simulink model "joint_sim_v1"  (R2018b)
settings: Solver=FixedStepAuto  StartTime=0.0  StopTime=8  FixedStep=0.001  MaxStep=0.001  RelTol=1e-3
undefined symbols (not defined in the file): alpha, D_el, F_c, F_s, J_joint, J_load, K_el, Kd_pos, Kd_trq, Kd_zf, Kp_pos, Kp_trq, Kp_zf, Ks_pos, Ks_trq, Ks_zf, Kt_pos, Kt_trq, Kt_zf, sigbuilder_block, sigma0, sigma1, sigma2, T_cur, T_signal_LPF, tau_max_ctrl, vs, X, Y, Z
libraries: sm_lib x6, nesl_utility x3, fcnLib4joint_sim x2, simulink x1
settings Model: Creator=l.ho  LastModifiedBy=qiming

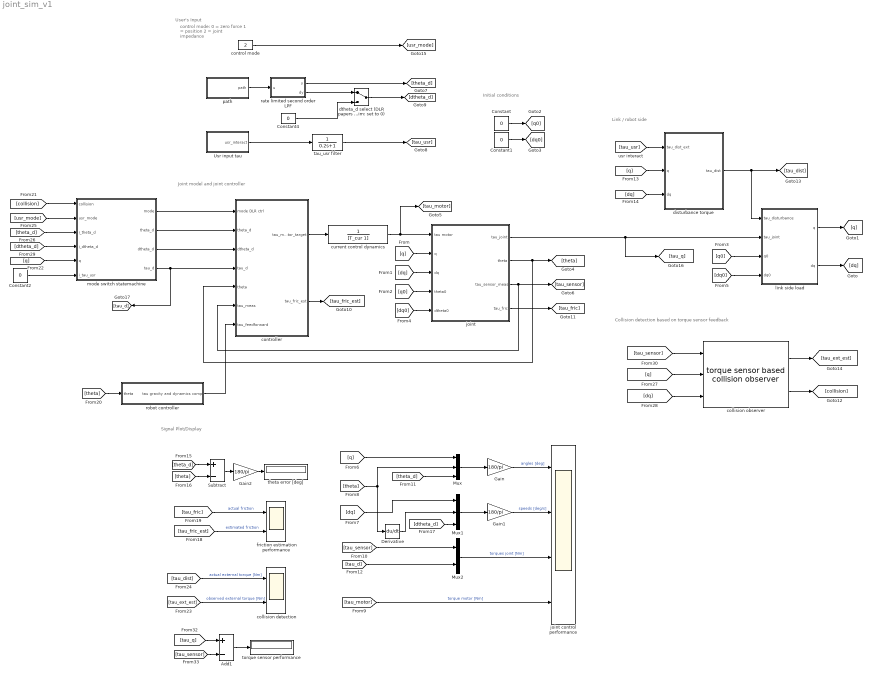
== system joint_sim_v1 ==
  note: Signal Plot/Display
  note: User's Input
  note: Collision detection based on torque sensor feedback
  note: Initial conditions
  note: Joint model and joint controller
  note: Link / robot side
  note: control mode:
      | 0 = zero force
      | 1 = position
      | 2 = joint impedance
  Add1 : Sum  Inputs=+-
  Constant{,1..2,4} (4 alike) : Constant  Value=0
  Derivative : Derivative
  Gain : Gain  Gain=180/pi
  Gain1 : Gain  Gain=180/pi
  Gain2 : Gain  Gain=180/pi
  Mux : Mux  Inputs=3
  Mux1 : Mux  Inputs=3
  Mux2 : Mux  Inputs=2
  Subtract : Sum  Inputs=+-
  Usr input tau : Subsystem  Tag=STV Subsys  LoadFcn=sigbuilder_block('load');  StartFcn=sigbuilder_block('start');  StopFcn=sigbuilder_block('stop');  ClipboardFcn=sigbuilder_block('clipboard');  mask(Sigbuilder block){tuvar=[0:10]}
      mask help: Simulink:masks:SigbuilderBlock_MD
      mask init:
      | if ~strcmp(get_param(bdroot(gcbh),'SimulationStatus'),'stopped') tuvar = sigbuilder_block('maskInit'); end
      settings: CopyFcn=sigbuilder_block('copy');  DeleteFcn=sigbuilder_block('delete');  ModelCloseFcn=sigbuilder_block('modelClose');  PreSaveFcn=sigbuilder_block('preSave');  PauseFcn=sigbuilder_block('pause');  ContinueFcn=sigbuilder_block('continue');  NameChangeFcn=sigbuilder_block('namechange');  OpenFcn=sigbuilder_block('open',[425.25 55.5 558 422.25 ]);  CloseFcn=sigbuilder_block('close');
      mask Display: plot(0, 0, 100, 100,[2, 2, 32, 32, 2], [68, 8, 8, 68, 68],[32, 2], [38, 38], [32, 19, 2],[53, 60, 44], [32, 17, 17, 2],[16, 16, 31, 31]);txt = getActiveGroup(gcbh);text(2, 100, txt,'verticalAlignment', 'top');
  "collision detection " : Scope  NumInputPorts=2
  "collision observer " : fcnLib4joint_sim/ torque sensor based collision observer   SystemSampleTime=-1
  control mode : Constant  Value=2
  controller : Subsystem
  current control dynamics : TransferFcn  Denominator=[T_cur 1]
  disturbance torque : Subsystem
  dtheta_d select (DLR papers and sim: set to 0) : ManualSwitch
  friction estimation performance : Scope  NumInputPorts=2
  joint : Subsystem
  joint control performance : Scope  NumInputPorts=4
  link side load : Subsystem
  mode switch statemachine : Stateflow chart  TreatAsAtomicUnit=on
  path : Subsystem  Tag=STV Subsys  LoadFcn=sigbuilder_block('load');  StartFcn=sigbuilder_block('start');  StopFcn=sigbuilder_block('stop');  ClipboardFcn=sigbuilder_block('clipboard');  mask(Sigbuilder block){tuvar=[0:10]}
      mask help: Simulink:masks:SigbuilderBlock_MD
      mask init:
      | if ~strcmp(get_param(bdroot(gcbh),'SimulationStatus'),'stopped') tuvar = sigbuilder_block('maskInit'); end
      settings: CopyFcn=sigbuilder_block('copy');  DeleteFcn=sigbuilder_block('delete');  ModelCloseFcn=sigbuilder_block('modelClose');  PreSaveFcn=sigbuilder_block('preSave');  PauseFcn=sigbuilder_block('pause');  ContinueFcn=sigbuilder_block('continue');  NameChangeFcn=sigbuilder_block('namechange');  OpenFcn=sigbuilder_block('open',[427.5 91.5 543 377.25 ]);  CloseFcn=sigbuilder_block('close');
      mask Display: plot(0, 0, 100, 100,[2, 2, 32, 32, 2], [68, 8, 8, 68, 68],[32, 2], [38, 38], [32, 19, 2],[53, 60, 44], [32, 17, 17, 2],[16, 16, 31, 31]);txt = getActiveGroup(gcbh);text(2, 100, txt,'verticalAlignment', 'top');
  rate limited second order LPF : Subsystem
  robot controller : Subsystem
  tau_usr filter : TransferFcn  Denominator=[0.2 1]
  theta error [deg] : Display
  torque sensor performance : Display
  wires:
  Constant/1 -> [q0]
  Constant1/1 -> [dq0]
  controller/1(tau_motor_target) -> current control dynamics/1
  joint/1(tau_joint) -> link side load/2(tau_joint), [tau_q]
  [dq0] -> link side load/4(dq0)
  [q0] -> link side load/3(q0)
  link side load/2(dq) -> [dq]
  link side load/1(q) -> [q]
  joint/2(theta) -> [theta], controller/5(theta)
  joint/3(tau_sensor_meas) -> controller/6(tau_meas), [tau_sensor]
  disturbance torque/1(tau_dist) -> [tau_dist], link side load/1(tau_disturbance)
  current control dynamics/1 -> [tau_motor], joint/1(tau motor)
  [theta] -> Mux/2, Derivative/1
  [q] -> Mux/1
  Mux/1 -> Gain/1
  Mux1/1 -> Gain1/1
  [dq] -> Mux1/1
  Derivative/1 -> Mux1/2
  [tau_sensor] -> Mux2/1
  Mux2/1 -> joint control performance/3  "torques joint [Nm]"
  [theta_d] -> Mux/3
  [tau_d] -> Mux2/2
  rate limited second order LPF/1(y) -> [theta_d]
  tau_usr filter/1 -> [tau_usr]
  [q] -> disturbance torque/2(q)
  [dq] -> disturbance torque/3(dq)
  Gain/1 -> joint control performance/1  "angles [deg]"
  Gain1/1 -> joint control performance/2  "speeds [deg/s]"
  [theta_d] -> Subtract/1
  [theta] -> Subtract/2
  Subtract/1 -> Gain2/1
  Gain2/1 -> theta error [deg]/1
  [dtheta_d] -> Mux1/3
  controller/2(tau_fric_est) -> [tau_fric_est]
  joint/4(tau_fric) -> [tau_fric]
  [tau_fric] -> friction estimation performance/1  "actual friction"
  [tau_fric_est] -> friction estimation performance/2  "estimated friction"
  [tau_motor] -> joint control performance/4  "torque motor [Nm]"
  rate limited second order LPF/2(dy) -> dtheta_d select (DLR papers and sim: set to 0)/1
  Constant4/1 -> dtheta_d select (DLR papers and sim: set to 0)/2
  [tau_ext_est] -> "collision detection "/2  "observed external torque [Nm]"
  [tau_dist] -> "collision detection "/1  "actual external torque [Nm]"
  [dq0] -> joint/5(dtheta0)
  [q] -> joint/2(q)
  [q0] -> joint/4(theta0)
  [dq] -> joint/3(dq)
  [q] -> "collision observer "/2
  "collision observer "/1 -> [tau_ext_est]
  [tau_sensor] -> "collision observer "/1
  [dq] -> "collision observer "/3
  "collision observer "/2 -> [collision]
  mode switch statemachine/1(mode) -> controller/1(mode DLR ctrl)
  mode switch statemachine/2(theta_d) -> controller/2(theta_d)
  mode switch statemachine/3(dtheta_d) -> controller/3(dtheta_d)
  dtheta_d select (DLR papers and sim: set to 0)/1 -> [dtheta_d]
  [q] -> mode switch statemachine/5(q)
  control mode/1 -> [usr_mode]
  [usr_mode] -> mode switch statemachine/2(usr_mode)
  [theta_d] -> mode switch statemachine/3(i_theta_d)
  [dtheta_d] -> mode switch statemachine/4(i_dtheta_d)
  Usr input tau/1(usr_interact) -> tau_usr filter/1
  mode switch statemachine/4(tau_d) -> [tau_d], controller/4(tau_d)
  robot controller/1(tau gravity and dynamics comp.) -> controller/7(tau_feedforward)
  [theta] -> robot controller/1(theta)
  [tau_usr] -> disturbance torque/1(tau_dist_ext)
  Constant2/1 -> mode switch statemachine/6(i_tau_usr)
  [tau_q] -> Add1/1
  [tau_sensor] -> Add1/2
  Add1/1 -> torque sensor performance/1
  path/1(path) -> rate limited second order LPF/1(u)
  [collision] -> mode switch statemachine/1(collision)

== system joint_sim_v1/Usr input tau ==
  Demux : Demux  Tag=STV Demux  Outputs=1
  FromWs : FromWorkspace  Tag=STV FromWs  VariableName=tuvar  SampleTime=0
      SigBuilderData=|
      | common.afterFinalStr = 'Extrapolate'
      | common.sampleTime = 0
      | dataSet.timeRange = [0 10]
      | dataSet.name = 'Group 1'
      | sbobj.Groups.Name = 'Group 1'
      | sbobj.Groups.Signals.Name = 'usr_interact'
      | sbobj.Groups.Signals.XData = [0 2 3 3 4 4 5 5 10]
      | sbobj.Groups.Signals.YData = [0 -0.002 -0.46 -0.455 -0.455 -0.45 0.002 0 0]
  usr_interact : Outport  Tag=STV Outport
  wires:
  FromWs/1 -> Demux/1
  Demux/1 -> usr_interact/1

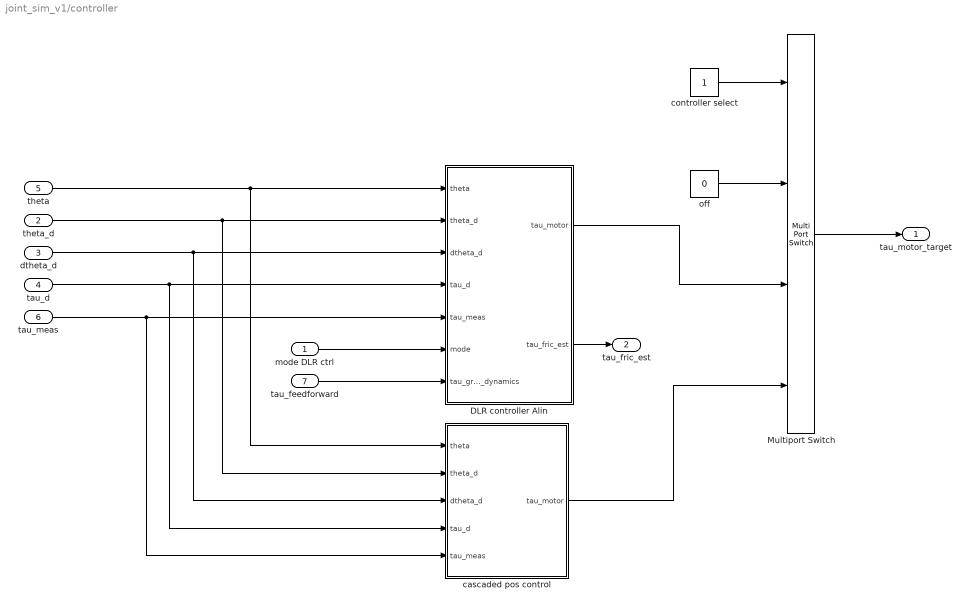
== system joint_sim_v1/controller ==
  mode DLR ctrl : Inport
  theta_d : Inport  Port=2
  dtheta_d : Inport  Port=3
  tau_d : Inport  Port=4
  theta : Inport  Port=5
  tau_meas : Inport  Port=6
  tau_feedforward : Inport  Port=7
  DLR controller Alin : Subsystem
  Multiport Switch : MultiPortSwitch  DataPortOrder=Zero-based contiguous  zeroidx=on
  cascaded pos control : Subsystem
  controller select : Constant
  off : Constant  Value=0
  tau_motor_target : Outport
  tau_fric_est : Outport  Port=2
  wires:
  Multiport Switch/1 -> tau_motor_target/1
  off/1 -> Multiport Switch/2
  controller select/1 -> Multiport Switch/1
  cascaded pos control/1(tau_motor) -> Multiport Switch/4
  theta/1 -> cascaded pos control/1(theta), DLR controller Alin/1(theta)
  theta_d/1 -> cascaded pos control/2(theta_d), DLR controller Alin/2(theta_d)
  tau_d/1 -> cascaded pos control/4(tau_d), DLR controller Alin/4(tau_d)
  DLR controller Alin/1(tau_motor) -> Multiport Switch/3
  mode DLR ctrl/1 -> DLR controller Alin/6(mode)
  tau_meas/1 -> DLR controller Alin/5(tau_meas), cascaded pos control/5(tau_meas)
  dtheta_d/1 -> cascaded pos control/3(dtheta_d), DLR controller Alin/3(dtheta_d)
  DLR controller Alin/2(tau_fric_est) -> tau_fric_est/1
  tau_feedforward/1 -> DLR controller Alin/7(tau_gravity_and_dynamics)

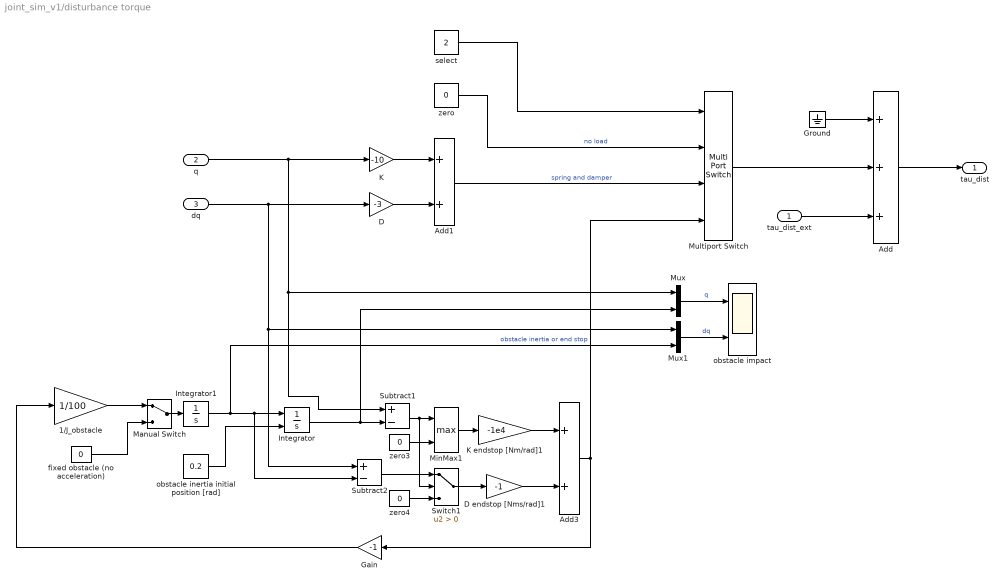
== system joint_sim_v1/disturbance torque ==
  tau_dist_ext : Inport
  q : Inport  Port=2
  dq : Inport  Port=3
  1/J_obstacle : Gain  Gain=1/100
  Add : Sum  Inputs=+++
  Add1 : Sum
  Add3 : Sum
  D : Gain  Gain=-3
  D endstop [Nms/rad]1 : Gain  Gain=-1
  Gain : Gain  Gain=-1
  Ground : Ground
  Integrator : Integrator  InitialConditionSource=external
  Integrator1 : Integrator
  K : Gain  Gain=-10
  K endstop [Nm/rad]1 : Gain  Gain=-1e4
  Manual Switch : ManualSwitch
  MinMax1 : MinMax  Function=max  Inputs=2
  Multiport Switch : MultiPortSwitch  DataPortOrder=Zero-based contiguous  zeroidx=on
  Mux : Mux  Inputs=2
  Mux1 : Mux  Inputs=2
  Subtract1 : Sum  Inputs=+-
  Subtract2 : Sum  Inputs=+-
  Switch1 : Switch  Criteria=u2 > Threshold
  fixed obstacle (no acceleration) : Constant  Value=0
  obstacle impact : Scope  NumInputPorts=2
  obstacle inertia initial position [rad] : Constant  Value=0.2
  select : Constant  Value=2
  zero : Constant  Value=0
  zero3 : Constant  Value=0
  zero4 : Constant  Value=0
  tau_dist : Outport
  wires:
  Add/1 -> tau_dist/1
  tau_dist_ext/1 -> Add/3
  Ground/1 -> Add/1
  Add1/1 -> Multiport Switch/3  "spring and damper"
  K/1 -> Add1/1
  D/1 -> Add1/2
  Multiport Switch/1 -> Add/2
  zero/1 -> Multiport Switch/2  "no load"
  select/1 -> Multiport Switch/1
  dq/1 -> D/1, Mux1/1, Subtract2/1
  zero4/1 -> Switch1/3
  D endstop [Nms/rad]1/1 -> Add3/2
  Switch1/1 -> D endstop [Nms/rad]1/1
  zero3/1 -> MinMax1/2
  MinMax1/1 -> K endstop [Nm/rad]1/1
  K endstop [Nm/rad]1/1 -> Add3/1
  Subtract1/1 -> MinMax1/1, Switch1/2
  Integrator/1 -> Mux/2, Subtract1/2
  Integrator1/1 -> Mux1/2, Subtract2/2, Integrator/1
  obstacle inertia initial position [rad]/1 -> Integrator/2
  Add3/1 -> Gain/1, Multiport Switch/4  "obstacle inertia or end stop"
  Gain/1 -> 1/J_obstacle/1
  Subtract2/1 -> Switch1/1
  q/1 -> Mux/1, Subtract1/1, K/1
  Mux/1 -> obstacle impact/1  "q"
  Mux1/1 -> obstacle impact/2  "dq"
  Manual Switch/1 -> Integrator1/1
  1/J_obstacle/1 -> Manual Switch/1
  fixed obstacle (no acceleration)/1 -> Manual Switch/2

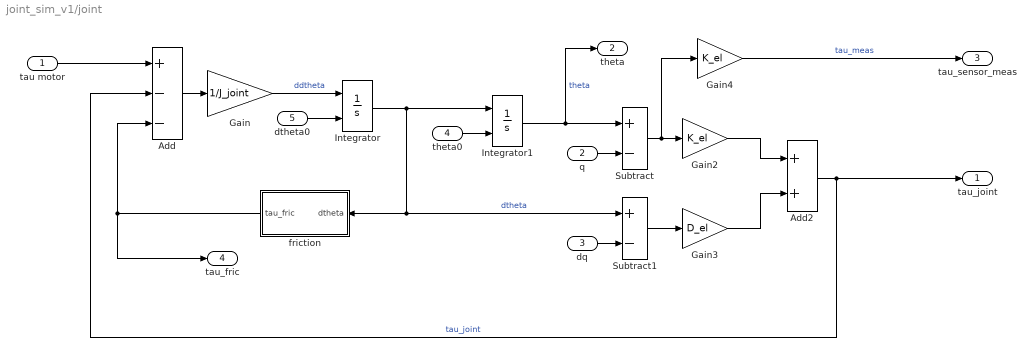
== system joint_sim_v1/joint ==
  tau motor : Inport
  q : Inport  Port=2
  dq : Inport  Port=3
  theta0 : Inport  Port=4
  dtheta0 : Inport  Port=5
  Add : Sum  Inputs=+--
  Add2 : Sum
  Gain : Gain  Gain=1/J_joint
  Gain2 : Gain  Gain=K_el
  Gain3 : Gain  Gain=D_el
  Gain4 : Gain  Gain=K_el
  Integrator : Integrator  InitialConditionSource=external
  Integrator1 : Integrator  InitialConditionSource=external
  Subtract : Sum  Inputs=+-
  Subtract1 : Sum  Inputs=+-
  friction : Subsystem
  tau_joint : Outport
  theta : Outport  Port=2
  tau_sensor_meas : Outport  Port=3
  tau_fric : Outport  Port=4
  wires:
  q/1 -> Subtract/2
  Gain4/1 -> tau_sensor_meas/1  "tau_meas"
  Gain/1 -> Integrator/1  "ddtheta"
  Gain3/1 -> Add2/2
  Gain2/1 -> Add2/1
  Add2/1 -> tau_joint/1, Add/2  "tau_joint"
  theta0/1 -> Integrator1/2
  Integrator/1 -> Integrator1/1, Subtract1/1, friction/1(dtheta)  "dtheta"
  Subtract/1 -> Gain4/1, Gain2/1
  Subtract1/1 -> Gain3/1
  tau motor/1 -> Add/1
  Add/1 -> Gain/1
  Integrator1/1 -> theta/1, Subtract/1  "theta"
  dtheta0/1 -> Integrator/2
  friction/1(tau_fric) -> tau_fric/1, Add/3
  dq/1 -> Subtract1/2

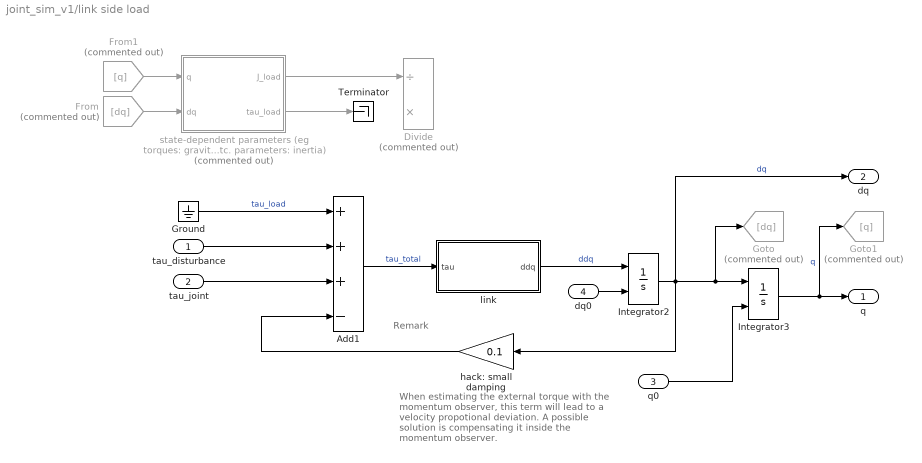
== system joint_sim_v1/link side load ==
  note: When estimating the external torque with the momentum observer, this term will lead to a velocity propotional deviation. A possible solution is compensating it inside the momentum observer.
  note: Remark
  tau_disturbance : Inport
  tau_joint : Inport  Port=2
  q0 : Inport  Port=3
  dq0 : Inport  Port=4
  Add1 : Sum  Inputs=+++-
  Divide : Product  Commented=on  Inputs=/*
  From : From  Commented=on  GotoTag=dq
  From1 : From  Commented=on  GotoTag=q
  Goto : Goto  Commented=on  GotoTag=dq
  Goto1 : Goto  Commented=on  GotoTag=q
  Ground : Ground
  Integrator2 : Integrator  InitialConditionSource=external
  Integrator3 : Integrator  InitialConditionSource=external
  Terminator : Terminator
  hack: small damping : Gain  Gain=0.1
  link : Subsystem
  "state-dependent parameters (eg torques: gravity, Coriolis, etc. parameters: inertia)" : Subsystem  Commented=on
  q : Outport
  dq : Outport  Port=2
  wires:
  tau_joint/1 -> Add1/3
  Integrator2/1 -> hack: small damping/1, dq/1, Goto/1, Integrator3/1  "dq"
  q0/1 -> Integrator3/2
  link/1(ddq) -> Integrator2/1  "ddq"
  tau_disturbance/1 -> Add1/2
  Add1/1 -> link/1(tau)  "tau_total"
  Integrator3/1 -> Goto1/1, q/1  "q"
  dq0/1 -> Integrator2/2
  "state-dependent parameters (eg torques: gravity, Coriolis, etc. parameters: inertia)"/2(tau_load) -> Terminator/1
  From/1 -> "state-dependent parameters (eg torques: gravity, Coriolis, etc. parameters: inertia)"/2(dq)
  From1/1 -> "state-dependent parameters (eg torques: gravity, Coriolis, etc. parameters: inertia)"/1(q)
  "state-dependent parameters (eg torques: gravity, Coriolis, etc. parameters: inertia)"/1(J_load) -> Divide/1
  hack: small damping/1 -> Add1/4
  Ground/1 -> Add1/1  "tau_load"

== system joint_sim_v1/path ==
  Demux : Demux  Tag=STV Demux  Outputs=1
  FromWs : FromWorkspace  Tag=STV FromWs  VariableName=tuvar  SampleTime=0
      SigBuilderData=|
      | common.afterFinalStr = 'Extrapolate'
      | common.sampleTime = 0
      | dataSet.timeRange = [0 10]
      | dataSet.name = 'Group 1'
      | sbobj.Groups.Name = 'Group 1'
      | sbobj.Groups.Signals.Name = 'path'
      | sbobj.Groups.Signals.XData = [0 10]
      | sbobj.Groups.Signals.YData = [0 0.88]
  path : Outport  Tag=STV Outport
  wires:
  FromWs/1 -> Demux/1
  Demux/1 -> path/1

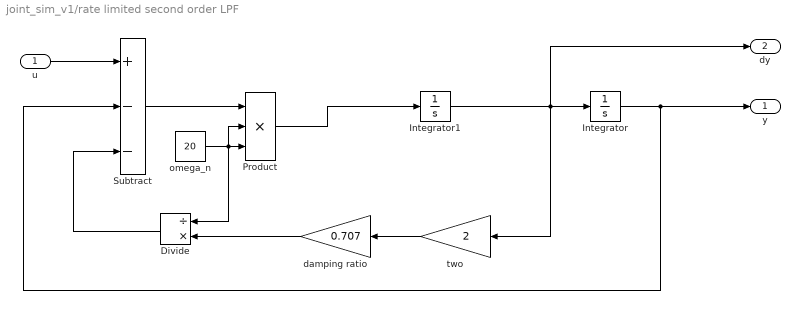
== system joint_sim_v1/rate limited second order LPF ==
  u : Inport
  Divide : Product  Inputs=/*
  Integrator : Integrator
  Integrator1 : Integrator  LimitOutput=on  UpperSaturationLimit=1  LowerSaturationLimit=-1
  Product : Product  Inputs=3
  Subtract : Sum  Inputs=+--
  damping ratio : Gain  Gain=0.707
  omega_n : Constant  Value=20
  two : Gain  Gain=2
  y : Outport
  dy : Outport  Port=2
  wires:
  Integrator1/1 -> two/1, dy/1, Integrator/1
  Integrator/1 -> Subtract/2, y/1
  u/1 -> Subtract/1
  Subtract/1 -> Product/1
  Product/1 -> Integrator1/1
  two/1 -> damping ratio/1
  Divide/1 -> Subtract/3
  omega_n/1 -> Divide/1, Product/2, Product/3
  damping ratio/1 -> Divide/2

== system joint_sim_v1/robot controller ==
  note: input list is still incomplete
  theta : Inport
  Ground : Ground
  Terminator : Terminator
  tau gravity and dynamics comp. : Outport
  wires:
  Ground/1 -> tau gravity and dynamics comp./1
  theta/1 -> Terminator/1

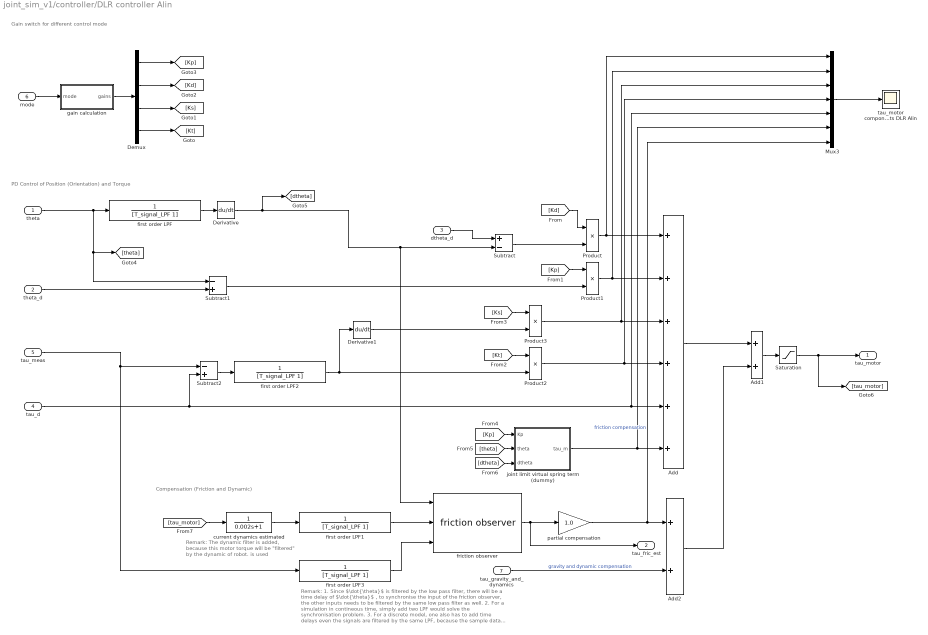
== system joint_sim_v1/controller/DLR controller Alin ==
  note: Remark:
      | The dynamic filter is added, because this motor torque will be "filtered" by the dynamic of robot.
      | is used
  note: Gain switch for different control mode
  note: PD Control of Position (Orientation) and Torque
  note: Compensation (Friction and Dynamic)
  note: Remark:
      | 1. Since $\dot{\theta}$ is filtered by the low pass filter, there will be a time delay of $\dot{\theta}$ ,
      | to synchronise the input of the friction observer, the other inputs needs to
      | be filtered by the same low pass filter as well.
      | 2. For a simulation in contineous time, simply add two LPF would solve
      | the synchronisation problem.
      | 3. For a discrete model, one also has to add time delays even the signals
      | are filtered by the same LPF, because the sample data used for derivation
      | could be taken several sample time later.
  theta : Inport
  theta_d : Inport  Port=2
  dtheta_d : Inport  Port=3
  tau_d : Inport  Port=4
  tau_meas : Inport  Port=5
  mode : Inport  Port=6
  tau_gravity_and_dynamics : Inport  Port=7
  Add : Sum  Inputs=++++++
  Add1 : Sum
  Add2 : Sum
  Demux : Demux
  Derivative : Derivative
  Derivative1 : Derivative
  Mux3 : Mux  Inputs=7
  Product{,1..3} (4 alike) : Product
  Saturation : Saturate  UpperLimit=tau_max_ctrl  LowerLimit=-tau_max_ctrl  LinearizeAsGain=off  ZeroCross=off
  Subtract : Sum  Inputs=+-
  Subtract1 : Sum  Inputs=-+
  Subtract2 : Sum  Inputs=-+
  current dynamics estimated : TransferFcn  Denominator=[0.002 1]
  first order LPF{,1..3} (4 alike) : TransferFcn  Denominator=[T_signal_LPF 1]
  friction observer : fcnLib4joint_sim/friction observer  SystemSampleTime=-1
  gain calculation : Subsystem
  joint limit virtual spring term (dummy) : Subsystem
  partial compensation : Gain  Gain=1.0
  tau_motor components DLR Alin : Scope
  tau_motor : Outport
  tau_fric_est : Outport  Port=2
  wires:
  Derivative1/1 -> Product3/2
  first order LPF2/1 -> Product2/2, Derivative1/1
  Product2/1 -> Mux3/4, Add/4
  Subtract/1 -> Product/2
  [Ks] -> Product3/1
  theta/1 -> [theta], Subtract1/1, first order LPF/1
  Add2/1 -> Add1/2
  partial compensation/1 -> Mux3/7, Add2/1  "friction compensation"
  Product/1 -> Mux3/1, Add/1
  joint limit virtual spring term (dummy)/1(tau_m) -> Mux3/6, Add/6
  tau_gravity_and_dynamics/1 -> Add2/2  "gravity and dynamic compensation"
  Product3/1 -> Mux3/3, Add/3
  first order LPF/1 -> Derivative/1
  Derivative/1 -> [dtheta], friction observer/1, Subtract/2
  [Kd] -> Product/1
  Saturation/1 -> [tau_motor], tau_motor/1
  dtheta_d/1 -> Subtract/1
  [Kp] -> joint limit virtual spring term (dummy)/1(Kp)
  Mux3/1 -> tau_motor components DLR Alin/1
  Product1/1 -> Mux3/2, Add/2
  Add/1 -> Add1/1
  [theta] -> joint limit virtual spring term (dummy)/2(theta)
  Subtract1/1 -> Product1/2
  Subtract2/1 -> first order LPF2/1
  [dtheta] -> joint limit virtual spring term (dummy)/3(dtheta)
  Add1/1 -> Saturation/1
  [Kt] -> Product2/1
  [Kp] -> Product1/1
  theta_d/1 -> Subtract1/2
  Demux/4 -> [Kt]
  Demux/2 -> [Kd]
  Demux/1 -> [Kp]
  Demux/3 -> [Ks]
  mode/1 -> gain calculation/1(mode)
  gain calculation/1(gains) -> Demux/1
  [tau_motor] -> current dynamics estimated/1
  current dynamics estimated/1 -> first order LPF1/1
  tau_meas/1 -> first order LPF3/1, Subtract2/1
  friction observer/1 -> partial compensation/1, tau_fric_est/1
  tau_d/1 -> Subtract2/2, Mux3/5, Add/5
  first order LPF1/1 -> friction observer/2
  first order LPF3/1 -> friction observer/3

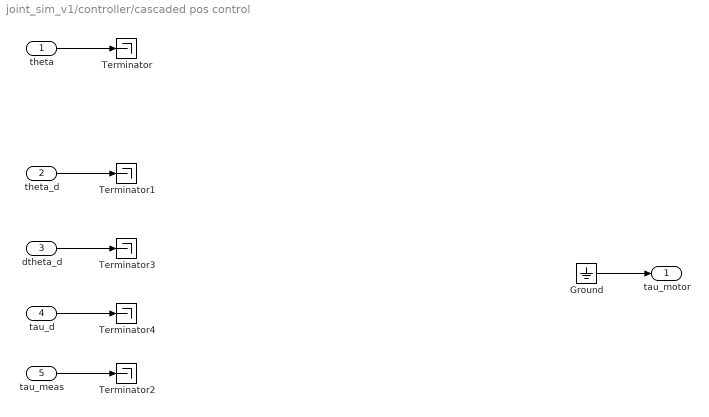
== system joint_sim_v1/controller/cascaded pos control ==
  theta : Inport
  theta_d : Inport  Port=2
  dtheta_d : Inport  Port=3
  tau_d : Inport  Port=4
  tau_meas : Inport  Port=5
  Ground : Ground
  Terminator{,1..4} (5 alike) : Terminator
  tau_motor : Outport
  wires:
  theta/1 -> Terminator/1
  theta_d/1 -> Terminator1/1
  tau_meas/1 -> Terminator2/1
  Ground/1 -> tau_motor/1
  dtheta_d/1 -> Terminator3/1
  tau_d/1 -> Terminator4/1

== system joint_sim_v1/joint/friction ==
  dtheta : Inport
  Add : Sum
  Compare To Constant : simulink/Logic and Bit Operations/Compare To Constant  relop=>=  const=0.01  OutDataTypeStr=boolean
  Constant : Constant  Value=F_c
  Gain4 : Gain  Gain=sigma2
  Subsystem : Subsystem
  tau_fric : Outport
  wires:
  dtheta/1 -> Subsystem/1(v), Gain4/1
  Gain4/1 -> Add/1  "viscous friction"
  Add/1 -> tau_fric/1
  Constant/1 -> Compare To Constant/1
  Compare To Constant/1 -> Subsystem/Enable
  Subsystem/1(F_fric dynamic) -> Add/2  "dynamic Stribeck friction"

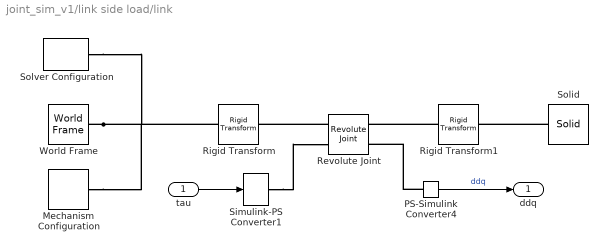
== system joint_sim_v1/link side load/link ==
  tau : Inport
  Mechanism Configuration : sm_lib/Utilities/Mechanism Configuration  UniformGravity=Constant  GravityVector=[0 0 -9.80665]  GravityUnits=m/s^2  LinearizationDelta=0.001
  PS-Simulink Converter4 : nesl_utility/PS-Simulink Converter  PhysicalDomain=network_engine_domain  SubClassName=ps_output  LeftPortType=input  RightPortType=output  PseudoPeriodic=off  Frequencies=[]  Unit=1  AffineConversion=off
  Revolute Joint : sm_lib/Joints/Revolute Joint  SenseConstraintForce=off  SenseConstraintForceX=off  SenseConstraintForceY=off  SenseConstraintForceZ=off  SenseConstraintTorque=off  SenseConstraintTorqueX=off  SenseConstraintTorqueY=off  SenseConstraintTorqueZ=off  SenseTotalForce=off  SenseTotalForceX=off  SenseTotalForceY=off  SenseTotalForceZ=off  SenseTotalTorque=off  SenseTotalTorqueX=off  SenseTotalTorqueY=off  SenseTotalTorqueZ=off  CompositeWrenchDir=FollowerOnBase  CompositeWrenchFrame=BaseFrame  EquilibriumPosition=0  EquilibriumPositionUnits=deg  SpringStiffness=0  SpringStiffnessUnits=N*m/deg  DampingCoefficient=0  DampingCoefficientUnits=N*m/(deg/s)  TorqueActuationMode=InputTorque  MotionActuationMode=ComputedMotion  SensePosition=off  SenseVelocity=off  SenseAcceleration=on  SenseTorqueForce=off  PositionTargetSpecify=off  PositionTargetPriority=High  PositionTargetValue=0  PositionTargetValueUnits=deg  VelocityTargetSpecify=off  VelocityTargetPriority=High  VelocityTargetValue=0  VelocityTargetValueUnits=deg/s
  Rigid Transform : sm_lib/Frames and Transforms/Rigid Transform  TranslationMethod=None  TranslationStandardOffset=150  TranslationLengthUnit=mm  TranslationStandardAxis=-X  TranslationCartesianOffset=[-150 0 0]  TranslationROffset=0  TranslationROffsetUnits=m  TranslationZOffset=0  TranslationZOffsetUnits=m  TranslationThetaOffset=0  TranslationThetaOffsetUnits=deg  RotationMethod=None  RotationAngleUnits=deg  RotationStandardAxis=+Z  RotationAngle=0.0  RotationArbitraryAxis=[0 0 1]  FollAlignAxisA=+X  BaseAlignAxisA=+Y  FollAlignAxisB=+Y  BaseAlignAxisB=+Z  RotationSequenceAxes=FollowerAxes  RotationSequence=XYX  RotationSequenceAngles=[0 0 0]  RotationSequenceAnglesUnits=deg  RotationMatrix=[1 0 0; 0 1 0; 0 0 1]
  Rigid Transform1 : sm_lib/Frames and Transforms/Rigid Transform  TranslationMethod=None  TranslationStandardOffset=150  TranslationLengthUnit=mm  TranslationStandardAxis=+X  TranslationCartesianOffset=[0 0 0]  TranslationROffset=0  TranslationROffsetUnits=m  TranslationZOffset=0  TranslationZOffsetUnits=m  TranslationThetaOffset=0  TranslationThetaOffsetUnits=deg  RotationMethod=None  RotationAngleUnits=deg  RotationStandardAxis=+Z  RotationAngle=0.0  RotationArbitraryAxis=[0 0 1]  FollAlignAxisA=+X  BaseAlignAxisA=+Y  FollAlignAxisB=+Y  BaseAlignAxisB=+Z  RotationSequenceAxes=FollowerAxes  RotationSequence=XYX  RotationSequenceAngles=[0 0 0]  RotationSequenceAnglesUnits=deg  RotationMatrix=[1 0 0; 0 1 0; 0 0 1]
  Simulink-PS Converter1 : nesl_utility/Simulink-PS Converter  PhysicalDomain=network_engine_domain  SubClassName=ps_input  LeftPortType=input  RightPortType=output  PseudoPeriodic=off  Frequencies=[]  NoiseDistribution=none  NoiseParameters=[]  Unit=1  AffineConversion=off  FilteringAndDerivatives=provide  SimscapeFilterOrder=1  InputFilterTimeConstant=0.001  UdotUserProvided=0
  Solid : sm_lib/Body Elements/Solid  InertiaType=Custom  Mass=1  MassUnits=kg  CenterOfMass=[0 0 0]  CenterOfMassUnits=m  MomentsOfInertia=[1 1 1.2252]  MomentsOfInertiaUnits=kg*m^2  ProductsOfInertia=[0 0 0]  ProductsOfInertiaUnits=kg*m^2  BasedOnType=Density  Density=2700  DensityUnits=kg/m^3  DoExposeReferenceFrame=on  SerializedFrames=<Frames/>  GraphicType=FromGeometry  MarkerShape=Sphere  MarkerSize=10  GraphicVisPropType=SimpleVisualProperties  GraphicDiffuseColor=[0.5 0.5 0.5]  GraphicSpecularColor=[0.5 0.5 0.5 1.0]  GraphicAmbientColor=[0.15 0.15 0.15 1.0]  GraphicEmissiveColor=[0.0 0.0 0.0 1.0]  GraphicShininess=75  GraphicOpacity=1.0  GeometryShape=Brick  RectangleSize=[1 1]  RectangleSizeUnits=m  BrickDimensions=[300 30 30]  BrickDimensionUnits=mm  CylinderRadius=1  CylinderRadiusUnits=m  CylinderLength=1  CylinderLengthUnits=m  SphereRadius=1  SphereRadiusUnits=m  EllipsoidRadii=[1 1 1]  EllipsoidRadiiUnits=m  ExtrusionCrossSection=[1 1; -1 1; -1 -1; 1 -1]  ExtrusionCrossSectionUnits=m  ExtrusionLength=1  ExtrusionLengthUnits=m  PolygonNumSides=3  PolygonOuterRadius=1  PolygonOuterRadiusUnits=m  ExtGeomFileType=STEP  ExtGeomFileUnits=m  RevolutionCrossSection=[1 1; 1 -1; 2 -1; 2 1]  RevolutionCrossSectionUnits=m  RevolutionExtent=Full  RevolutionAngle=180  RevolutionAngleUnits=deg
  Solver Configuration : nesl_utility/Solver Configuration  PhysicalDomain=network_engine_domain  SubClassName=solver  LeftPortType=input  RightPortType=generic  Tones=[]  Harmonics=[]  SimulateNoise=off  Profile=off  UseLocalSampling=off  EnableSwitchedLinearOptims=on  FrequencyDomain=off  UseCCode=off  RelTol=0.001  AbsTol=1e-06  MinStep=1e-09  ToWorkspace=off  RevertToSquareIcSolve=off  NumHomotopyIterations=100  PhasorMode=off  PhasorModeNumHarmonics=1  DoDC=off  ResidualTolerance=1e-09  UseLocalSolver=off  LocalSolverChoice=NE_BACKWARD_EULER_ADVANCER  LocalSolverSampleTime=0.001  DoFixedCost=off  MaxNonlinIter=3  MaxModeIter=2  LinearAlgebra=auto  EquationFormulation=NE_TIME_EF  DelaysMemoryBudget=1024  AutomaticFiltering=on  FilteringTimeConstant=0.001  PartitionStorageMethod=AS_NEEDED  PartitionMemoryBudget=1024
  World Frame : sm_lib/Frames and Transforms/World Frame
  ddq : Outport
  wires:
  tau/1 -> Simulink-PS Converter1/1
  PS-Simulink Converter4/1 -> ddq/1  "ddq"
  connections:
  World Frame/RConn1 -- Rigid Transform/LConn1 -- Solver Configuration/RConn1 -- Mechanism Configuration/RConn1
  Simulink-PS Converter1/RConn1 -- Revolute Joint/LConn2
  Revolute Joint/LConn1 -- Rigid Transform/RConn1
  Solid/RConn1 -- Rigid Transform1/RConn1
  PS-Simulink Converter4/LConn1 -- Revolute Joint/RConn2
  Rigid Transform1/LConn1 -- Revolute Joint/RConn1

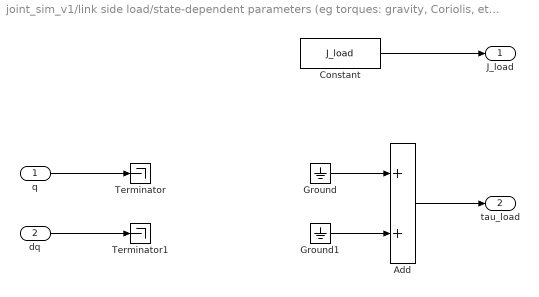
== system joint_sim_v1/link side load/state-dependent parameters (eg torques: gravity, Coriolis, etc. parameters: inertia) ==
  q : Inport
  dq : Inport  Port=2
  Add : Sum
  Constant : Constant  Value=J_load
  Ground : Ground
  Ground1 : Ground
  Terminator : Terminator
  Terminator1 : Terminator
  J_load : Outport
  tau_load : Outport  Port=2
  wires:
  Add/1 -> tau_load/1
  q/1 -> Terminator/1
  dq/1 -> Terminator1/1
  Ground/1 -> Add/1
  Ground1/1 -> Add/2
  Constant/1 -> J_load/1

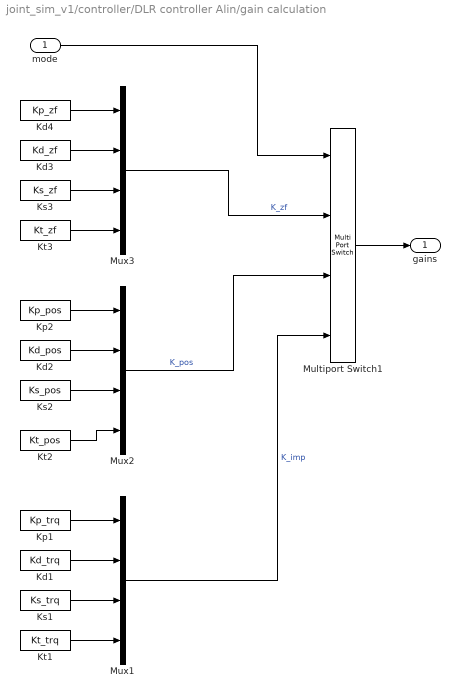
== system joint_sim_v1/controller/DLR controller Alin/gain calculation ==
  mode : Inport
  Kd1 : Constant  Value=Kd_trq
  Kd2 : Constant  Value=Kd_pos
  Kd3 : Constant  Value=Kd_zf
  Kd4 : Constant  Value=Kp_zf
  Kp1 : Constant  Value=Kp_trq
  Kp2 : Constant  Value=Kp_pos
  Ks1 : Constant  Value=Ks_trq
  Ks2 : Constant  Value=Ks_pos
  Ks3 : Constant  Value=Ks_zf
  Kt1 : Constant  Value=Kt_trq
  Kt2 : Constant  Value=Kt_pos
  Kt3 : Constant  Value=Kt_zf
  Multiport Switch1 : MultiPortSwitch  DataPortOrder=Zero-based contiguous  DiagnosticForDefault=None  zeroidx=on
  Mux1 : Mux
  Mux2 : Mux
  Mux3 : Mux
  gains : Outport
  wires:
  Kt1/1 -> Mux1/4
  Kd2/1 -> Mux2/2
  mode/1 -> Multiport Switch1/1
  Mux1/1 -> Multiport Switch1/4  "K_imp"
  Kp1/1 -> Mux1/1
  Kt2/1 -> Mux2/4
  Mux2/1 -> Multiport Switch1/3  "K_pos"
  Kd1/1 -> Mux1/2
  Ks2/1 -> Mux2/3
  Ks1/1 -> Mux1/3
  Kp2/1 -> Mux2/1
  Multiport Switch1/1 -> gains/1
  Mux3/1 -> Multiport Switch1/2  "K_zf"
  Kd4/1 -> Mux3/1
  Kd3/1 -> Mux3/2
  Kt3/1 -> Mux3/4
  Ks3/1 -> Mux3/3

== system joint_sim_v1/controller/DLR controller Alin/joint limit virtual spring term (dummy) ==
  Kp : Inport
  theta : Inport  Port=2
  dtheta : Inport  Port=3
  Ground : Ground
  Terminator : Terminator
  Terminator1 : Terminator
  Terminator2 : Terminator
  tau_m : Outport
  wires:
  Ground/1 -> tau_m/1
  dtheta/1 -> Terminator2/1
  Kp/1 -> Terminator/1
  theta/1 -> Terminator1/1

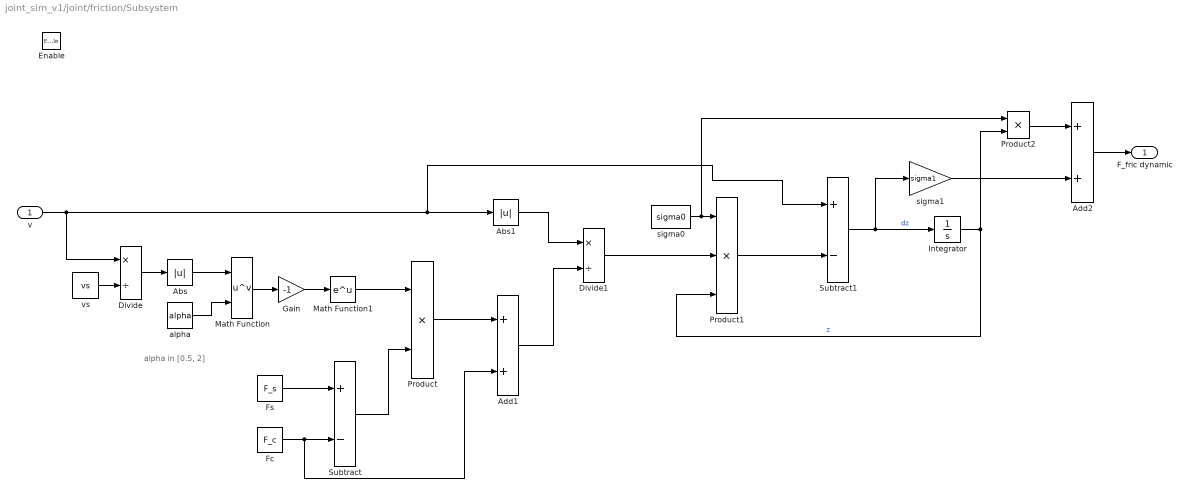
== system joint_sim_v1/joint/friction/Subsystem ==
  note: alpha in [0.5, 2]
  v : Inport
  Enable : EnablePort  StatesWhenEnabling=reset
  Abs : Abs
  Abs1 : Abs
  Add1 : Sum
  Add2 : Sum
  Divide : Product  Inputs=*/
  Divide1 : Product  Inputs=*/
  Fc : Constant  Value=F_c
  Fs : Constant  Value=F_s
  Gain : Gain  Gain=-1
  Integrator : Integrator
  Math Function : Math  Operator=pow  SaturateOnIntegerOverflow=on
  Math Function1 : Math  SaturateOnIntegerOverflow=on
  Product : Product
  Product1 : Product  Inputs=3
  Product2 : Product
  Subtract : Sum  Inputs=+-
  Subtract1 : Sum  Inputs=+-
  alpha : Constant  Value=alpha
  sigma0 : Constant  Value=sigma0
  sigma1 : Gain  Gain=sigma1
  vs : Constant  Value=vs
  F_fric dynamic : Outport  OutputWhenDisabled=reset  InitialOutput=0
  wires:
  Product1/1 -> Subtract1/2
  Divide1/1 -> Product1/2
  Abs/1 -> Math Function/1
  sigma1/1 -> Add2/2
  sigma0/1 -> Product2/1, Product1/1
  v/1 -> Subtract1/1, Abs1/1, Divide/1
  Product2/1 -> Add2/1
  Product/1 -> Add1/1
  Subtract/1 -> Product/2
  Math Function1/1 -> Product/1
  Divide/1 -> Abs/1
  alpha/1 -> Math Function/2
  Integrator/1 -> Product2/2, Product1/3  "z"
  Gain/1 -> Math Function1/1
  Fc/1 -> Add1/2, Subtract/2
  vs/1 -> Divide/2
  Subtract1/1 -> sigma1/1, Integrator/1  "dz"
  Math Function/1 -> Gain/1
  Add1/1 -> Divide1/2
  Abs1/1 -> Divide1/1
  Fs/1 -> Subtract/1
  Add2/1 -> F_fric dynamic/1

== stateflow chart joint_sim_v1/mode switch statemachine ==
  state Usr_defined_mode
    en:
    mode = usr_mode;
    du:
    theta_d = i_theta_d;
    dtheta_d = i_dtheta_d;
    tau_d = i_tau_usr
    state Position_control
    state Impedance_control
    state Zero_force_control
    (default) -> Position_control
    (junction 37) -> Position_control [order 3] : [usr_mode == 1]
    (junction 37) -> Impedance_control [order 2] : [usr_mode == 2]
    Usr_defined_mode -> (junction 37) [order 1]
    (junction 37) -> Zero_force_control [order 1] : [usr_mode == 0]
  state Collision_mode
    en:
    mode = 2;
    theta_d = max(q - pi/6, 0);
    dtheta_d = 0;
  (default) -> Usr_defined_mode
  Usr_defined_mode -> Collision_mode [order 1] : [collision == 1]
  data: collision input; mode output; usr_mode input; i_theta_d input; i_dtheta_d input; theta_d output; dtheta_d output; q input; tau_d output; i_tau_usr input
